simulink model "EuroNCAP_PedAEB"  (R2014b)
settings: Solver=ode45  SolverMode=SingleTasking  StartTime=0.0  StopTime=100  RelTol=1e-3
libraries: Solver_SF x1
settings Model: Creator=elowe  LastModifiedBy=elowe
settings OptimizationCC: BlockReduction=off  BooleanDataType=off
settings DebuggingCC: SaveWithParameterizedLinksMsg=none  UnderspecifiedInitializationDetection=Classic  MergeDetectMultiDrivingBlocksExec=none  SignalResolutionControl=TryResolveAllWithWarning  SolverPrmCheckMsg=none
settings HardwareCC: TargetUnknown=on

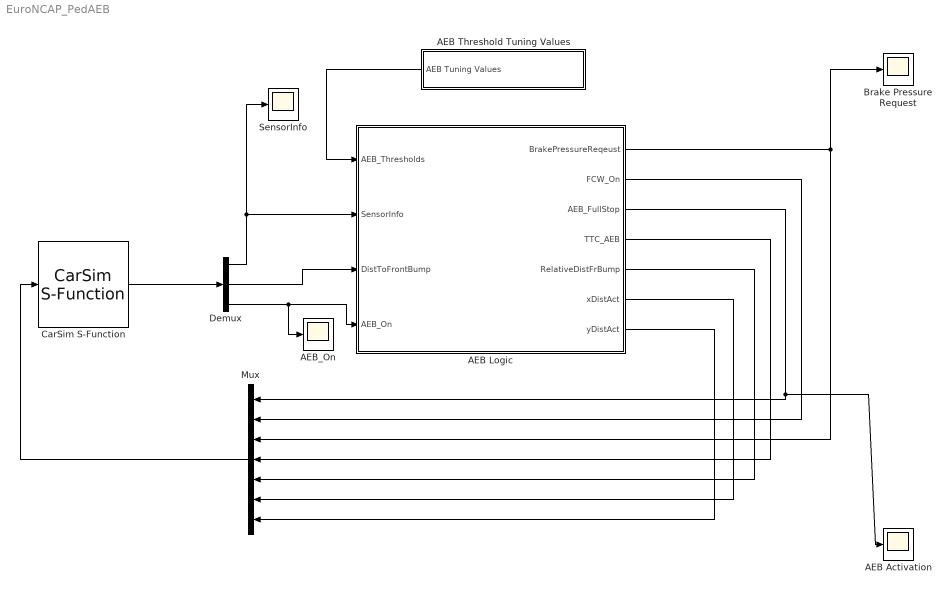
== system EuroNCAP_PedAEB ==
  AEB Activation : Scope
      settings: YMin=-0.06941  YMax=1.10847  SaveName=ScopeData6
  AEB Logic : MATLAB Function  TreatAsAtomicUnit=on
  AEB Threshold Tuning Values : Subsystem
  AEB_On : Scope
      settings: YMin=-0.125  YMax=1.125
  Brake Pressure Request : Scope
      settings: YMin=-0.625  YMax=5.625  SaveName=ScopeData5
  CarSim S-Function : Solver_SF/CarSim S-Function  Priority=1  SIMFILE=simfile.sim  Run_RTs=off  vs_state_ind=Run  StopMode_ind=Vehicle Model
  Demux : Demux  Outputs=[6 1 1]
  Mux : Mux  Inputs=7
  SensorInfo : Scope
      settings: ShowLegends=on  YMin=-23.16129  YMax=56
  wires:
  AEB Threshold Tuning Values/1(AEB Tuning Values) -> AEB Logic/1(AEB_Thresholds)
  AEB Logic/1(BrakePressureReqeust) -> Brake Pressure Request/1, Mux/3
  AEB Logic/2(FCW_On) -> Mux/2
  Demux/1 -> SensorInfo/1, AEB Logic/2(SensorInfo)
  Demux/2 -> AEB Logic/3(DistToFrontBump)
  AEB Logic/3(AEB_FullStop) -> AEB Activation/1, Mux/1
  Demux/3 -> AEB_On/1, AEB Logic/4(AEB_On)
  AEB Logic/4(TTC_AEB) -> Mux/4
  AEB Logic/5(RelativeDistFrBump) -> Mux/5
  Mux/1 -> CarSim S-Function/1
  CarSim S-Function/1 -> Demux/1
  AEB Logic/6(xDistAct) -> Mux/6
  AEB Logic/7(yDistAct) -> Mux/7

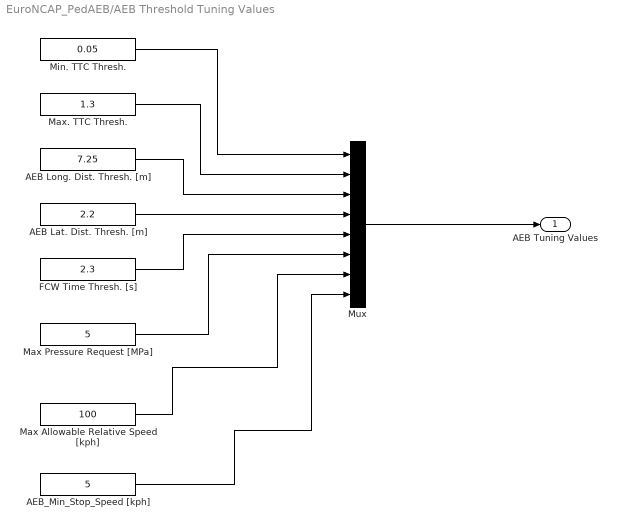
== system EuroNCAP_PedAEB/AEB Threshold Tuning Values ==
  AEB Lat. Dist. Thresh. [m] : Constant  Value=2.2
  AEB Long. Dist. Thresh. [m] : Constant  Value=7.25
  AEB_Min_Stop_Speed [kph] : Constant  Value=5
  FCW Time Thresh. [s] : Constant  Value=2.3
  Max Allowable Relative Speed [kph] : Constant  Value=100
  Max Pressure Request [MPa] : Constant  Value=5
  Max. TTC Thresh. : Constant  Value=1.3
  Min. TTC Thresh. : Constant  Value=0.05
  Mux : Mux  Inputs=8
  AEB Tuning Values : Outport
  wires:
  FCW Time Thresh. [s]/1 -> Mux/5
  Max. TTC Thresh./1 -> Mux/2
  AEB Lat. Dist. Thresh. [m]/1 -> Mux/4
  AEB Long. Dist. Thresh. [m]/1 -> Mux/3
  Mux/1 -> AEB Tuning Values/1
  Min. TTC Thresh./1 -> Mux/1
  Max Pressure Request [MPa]/1 -> Mux/6
  Max Allowable Relative Speed [kph]/1 -> Mux/7
  AEB_Min_Stop_Speed [kph]/1 -> Mux/8

== matlab function EuroNCAP_PedAEB/AEB Logic ==
  data: AEB_Thresholds input; BrakePressureReqeust output; FCW_On output; SensorInfo input; DistToFrontBump input; AEB_FullStop output; AEB_On input; TTC_AEB output; RelativeDistFrBump output; xDistAct output; yDistAct output
function [BrakePressureReqeust, FCW_On, AEB_FullStop,...
    TTC_AEB, RelativeDistFrBump, xDistAct, ...
    yDistAct] = AEB_SystemOutputs(AEB_Thresholds,...
    SensorInfo, DistToFrontBump, AEB_On)

TTC_minTimeThresh = AEB_Thresholds(1); %both time and distance minimum 
% threshold value
TTC_maxTimeThresh = AEB_Thresholds(2);
AEB_longDistThresh = AEB_Thresholds(3);
AEB_latDistThresh = AEB_Thresholds(4);
FCW_timeThresh = AEB_Thresholds(5);
MaxPressureReq = AEB_Thresholds(6);
AEB_MaxAllowRelSpeed = AEB_Thresholds(7);
AEB_Min_Stop_Speed = AEB_Thresholds(8);

relDist = SensorInfo(1); % [m]: relative distance between the camera  
% and the detected object
relSpeed = SensorInfo(2); % [km/h]: relative speed between the camera 
% sensor and the object detected
relBearing = SensorInfo(3); % [deg] relative bearing between the camera 
% sensor and the detected object 
objHeight = SensorInfo(4); % [m] vertical distance between the cameara
% sensor and the detected object 
cameraObjDetect =  SensorInfo(5); % [-] boolean for when an object is 
% detected by the camera sensor
currentVehX_Speed =  SensorInfo(6); % [km/h] current longitudinal speed of
% ego vehicle in the global reference frame

minDistThresh = TTC_minTimeThresh; % [m] Minimum distance threshold
distCamToFrBumper = DistToFrontBump; % [m] this is the known longitudinal 
% distance from the front bumper to the camera sensor 

FCW_On = 0;

xDistAct = 0; % [m] longitudinal distance from the front bumper
yDistAct = 0; % [m] lateral distance from the front bumper
heightAngle = 0; % [deg] vertical angle of the target center from the 
% camera origin
xyDistSens = 0; % [m] relative distance resolved in the x-y plane

relBearFrtBump = 0; % [rad]
relDistFrtBump = 0; % [m] relative distance from the front bumper along 
% the vehicle longitudinal axis, to the obstacle
RelativeDistFrBump = 0; % [m] output value, equivalent to relDistFrtBump

TTC_AEB = 0; % TTC calculation value [s]
AEB_TimeBool = 0; % boolean to know if AEB time threshold has been 
% satisfied for activation
AEB_DistBool = 0; % boolean to know if AEB distance threshold has been 
% satisfied for activation
AEB_FullStop = 0; % boolean for activating AEB, at maximum braking
FCW_On = 0; % boolean for activating FCW or not
RelSpeedOk = 0; % [km/h] relative speed with saturation protection, for the
% point of initial detection by the sensor
if cameraObjDetect >= 1 
    if abs(relDist) > 0
        heightAngle = asin(objHeight/relDist);
    else
        heightAngle = 0;
    end
    xyDistSens = relDist*cos(heightAngle); % resolve 3D relative distance
    % vector into the x-y plane
    xDistAct = xyDistSens*cos(relBearing*(pi/180))-distCamToFrBumper;
    yDistAct =  xyDistSens*sin(relBearing*(pi/180));
else
    heightAngle = 0;
    xyDistSens = 0;
    xDistAct = 0;
    yDistAct =  0;
end

if abs(yDistAct) > minDistThresh
    relBearFrtBump = atan(yDistAct/xDistAct);
else
    relBearFrtBump = 0;
end

if abs(relBearFrtBump) > 0
    relDistFrtBump = yDistAct/sin(relBearFrtBump); 
    RelativeDistFrBump = relDistFrtBump;
else
    relDistFrtBump = 0;
    RelativeDistFrBump = relDistFrtBump;
end
if ( abs(relSpeed) < AEB_MaxAllowRelSpeed)
    RelSpeedOk = relSpeed;
else
    RelSpeedOk = 0;
end

% Time to collision from object to the ego vehicle's front bumper
if ( RelSpeedOk < -TTC_minTimeThresh) && (cameraObjDetect >= 1)
    TTC_AEB =  abs(relDistFrtBump/(relSpeed/3.6));
else
    TTC_AEB =  0;
end
% TTC time threshold condition
if (TTC_AEB < TTC_maxTimeThresh) && (TTC_AEB > TTC_minTimeThresh) && ...
        abs(yDistAct)
    AEB_TimeBool = 1;
else
    AEB_TimeBool = 0;
end
% TTC distance threshold condition
if (xDistAct < AEB_longDistThresh) && ...
        (abs(yDistAct) < AEB_latDistThresh)
    AEB_DistBool = 1;
else
    AEB_DistBool = 0;
end

%*********************** AEB activation ***********************
if (cameraObjDetect >= 1)   % only apply AEB if the object is detected by 
                            % the camera sensor
    if (AEB_On == 1) && ((AEB_TimeBool == 1) || (AEB_DistBool == 1) ...
            || abs(currentVehX_Speed) < AEB_Min_Stop_Speed)
        AEB_FullStop = 1;
    else
        AEB_FullStop = 0; 
    end
end
BrakePressureReqeust = MaxPressureReq*AEB_FullStop;
%*********************** FCW activation ***********************
if (cameraObjDetect >= 1) && (relSpeed < 0) && (TTC_AEB < FCW_timeThresh)...
        && (abs(yDistAct) < AEB_latDistThresh)
    FCW_On = 1;
elseif AEB_FullStop == 1
    FCW_On = 1;
else
    FCW_On = 0;
end
